simulink model "CrazyPendulum"  (Simulink 7.9)
settings: Solver=ode45  StartTime=0.0  StopTime=10  RelTol=1e-3
libraries: vrlib x2
settings Model: Creator=karo  LastModifiedBy=karo

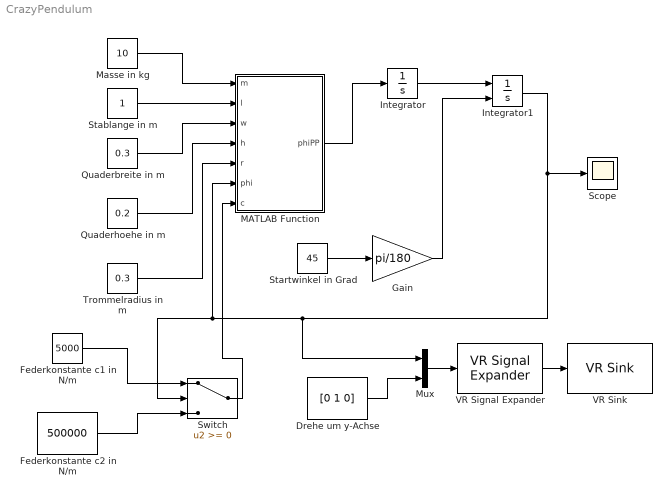
== system CrazyPendulum ==
  Drehe um y-Achse : Constant  Value=[0 1 0]
  Federkonstante c1 in N/m : Constant  Value=5000
  Federkonstante c2 in N/m : Constant  Value=500000
  Gain : Gain  Gain=pi/180
  Integrator : Integrator
  Integrator1 : Integrator  InitialConditionSource=external
  MATLAB Function : MATLAB Function  TreatAsAtomicUnit=on
  Masse in kg : Constant  Value=10
  Mux : Mux  Inputs=2
  Quaderbreite in m : Constant  Value=0.3
  Quaderhoehe in m : Constant  Value=0.2
  Scope : Scope
  Stablange in m : Constant
  Startwinkel in Grad : Constant  Value=45
  Switch : Switch
  Trommelradius in m : Constant  Value=0.3
  VR Signal Expander : vrlib/VR Signal Expander  outwidth=4  outidx=[4 1 2 3]
  VR Sink : vrlib/VR Sink  SampleTime=0.005  ViewEnable=on  RemoteChange=off  RemoteView=off  FieldsWritten=Seiltrommel.rotation.4.1.1.double  WorldFileName=CrazyPendlm.wrl  AutoView=off  VideoDimensions=[]  AllowVariableSize=off
  wires:
  Integrator/1 -> Integrator1/1
  Masse in kg/1 -> MATLAB Function/1(m)
  Stablange in m/1 -> MATLAB Function/2(l)
  Quaderbreite in m/1 -> MATLAB Function/3(w)
  Quaderhoehe in m/1 -> MATLAB Function/4(h)
  Trommelradius in m/1 -> MATLAB Function/5(r)
  Startwinkel in Grad/1 -> Gain/1
  Federkonstante c2 in N/m/1 -> Switch/3
  Federkonstante c1 in N/m/1 -> Switch/1
  Integrator1/1 -> Scope/1, MATLAB Function/6(phi), Switch/2, Mux/1
  Gain/1 -> Integrator1/2
  MATLAB Function/1(phiPP) -> Integrator/1
  Switch/1 -> MATLAB Function/7(c)
  Drehe um y-Achse/1 -> Mux/2
  Mux/1 -> VR Signal Expander/1
  VR Signal Expander/1 -> VR Sink/1

== matlab function MATLAB Function ==
  data: m input double; phiPP output double; l input double; w input double; h input double; r input double; phi input double; c input double
function phiPP = fcn(m, l, w, h, r, phi, c)

g = -9.81;  % Beschleinigung durch Gravitation
FG = m * g; % Gravitationskraft
MG = FG * sin(phi) * (l + h/2); % Drehmoment des Pendels

s = phi * r;    % Auslenkung
FF = c * s;     % Federkraft
MF = FF * r;    % Drehmoment der Feder

JS = 1/12 * m * (w^2 + h^2);    % Massentraegheitsmoments des Quaders
JA = JS + m * (l + h/2)^2;      % Mass.tr.moment nach Satz von Steiner

phiPP = (MG - MF)/JA;
